simulink model "testsonar"  (R2021b)
settings: Solver=FixedStepAuto  StartTime=0.0  StopTime=inf  FixedStep=1/10  RelTol=1e-3
libraries: robotlib x2
settings Model: Creator=lamarre  LastModifiedBy=lamarre
settings OptimizationCC: EnhancedBackFolding=on  PassReuseOutputArgsAs=Individual arguments  ZeroExternalMemoryAtStartup=off  ZeroInternalMemoryAtStartup=off  MaxStackSize=64  OptimizeBlockOrder=speed  DifferentSizesBufferReuse=on  OptimizationCustomize=off  EfficientTunableParamExpr=on
settings DebuggingCC: ParameterTunabilityLossMsg=error
settings HardwareCC: ProdBitPerPointer=32  ProdBitPerSizeT=32  ProdBitPerPtrDiffT=32  ProdLargestAtomicFloat=None  ProdIntDivRoundTo=Undefined  ProdEndianess=Unspecified  ProdWordSize=32  ProdHWDeviceType=Generic->Unspecified (assume 32-bit Generic)
settings SFSimCC: MATLABDynamicMemAlloc=off
settings RTWCC: Description=Embedded Coder  SystemTargetFile=ert.tlc  HardwareBoard=Robot Operating System (ROS)  TLCOptions="-aInlineSetEventsForThisBaseRateFcn=TLC_FALSE -aSuppressMultiTaskScheduler=TLC_FALSE  -aRateBasedStepFcn=0"  TemplateMakefile=ert_default_tmf  Toolchain=Catkin  TargetLang=C++
settings CodeAppCC: ForceParamTrailComments=on  IgnoreCustomStorageClasses=off  OperatorAnnotations=on  SimulinkDataObjDesc=on  SFDataObjDesc=on  InsertBlockDesc=on

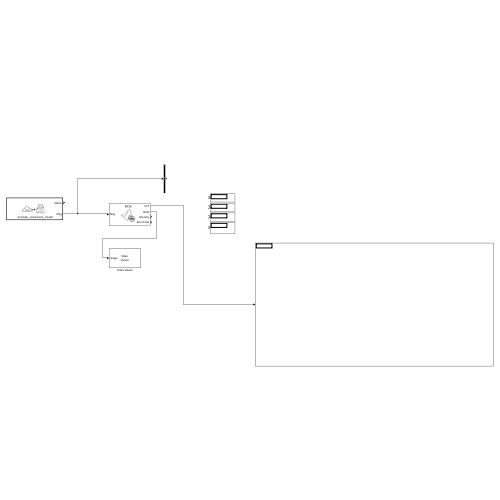
[thumbnail: Simulink's stored preview of the top-level diagram]
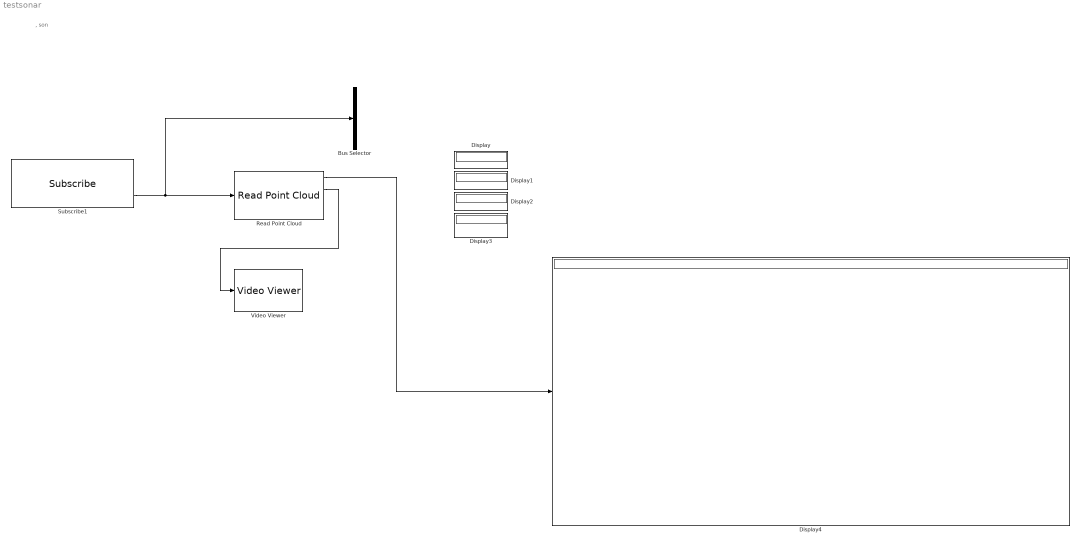
== system testsonar ==
  note: , son
  Bus Selector : BusSelector  OutputSignals=Data
  Display{,1..4} (5 alike) : Display
  Read Point Cloud : robotlib/Read Point Cloud  MaximumPointCloudSize=[1, 137856]  PreserveStructure=off  ShowRGBOutput=on  ShowIntensityOutput=on  ShowErrorCodeOutput=on  VariableSizeOutputs=off
      settings: SourceProductBaseCode=RR
  Subscribe1 : robotlib/Subscribe  topicSource=Specify your own  topic=/provider_sonar/point_cloud2  messageType=sensor_msgs/PointCloud2  SampleTime=-1  legacyBusStruct=off  messageQueueLength=1
  Video Viewer : VideoViewer  FigPos=[73 1078 1861 942]
  wires:
  Subscribe1/2 -> Bus Selector/1, Read Point Cloud/1
  Read Point Cloud/2 -> Video Viewer/1
  Read Point Cloud/1 -> Display4/1
